simulink model "Lora_os_all_16M64M_bw500sf12"  (R2022b)
settings: Solver=FixedStepDiscrete  StartTime=0.0  StopTime=0.06  RelTol=1e-3
undefined symbols (not defined in the file or in its folder): cr, crc, fs, has_header, ldr, payload, preamble_len, sf
libraries: hdlsllib x4, simulink x2
settings Model: DataTypeOverride=Off  Creator=28627  LastModifiedBy=X_Ditto
settings SolverCC: AlgebraicLoopSolver=TrustRegion
settings DataIOCC: SaveOutput=off  SaveTime=off
settings OptimizationCC: BlockReduction=off  ConditionallyExecuteInputs=off  DefaultParameterBehavior=Inlined
settings DebuggingCC: AlgebraicLoopMsg=error  SingleTaskRateTransMsg=error  UnconnectedInputMsg=warning  UnconnectedOutputMsg=warning  UnconnectedLineMsg=warning  StrictBusMsg=ErrorOnBusTreatedAsVector  SFMachineParentedDataDiag=warning  ArithmeticOperatorsInVariantConditions=warning
settings HardwareCC: ProdBitPerPointer=32  ProdBitPerSizeT=32  ProdBitPerPtrDiffT=32  ProdLargestAtomicFloat=None  ProdIntDivRoundTo=Undefined  ProdEndianess=Unspecified  ProdWordSize=32  ProdHWDeviceType=ASIC/FPGA->ASIC/FPGA  ProdEqTarget=off
settings ModelReferenceCC: EnableRefExpFcnMdlSchedulingChecks=on
settings SFSimCC: SimUseLocalCustomCode=off  CustomCodeUndefinedFunction=UseInterfaceOnly
settings RTWCC: RTWUseLocalCustomCode=off
settings CodeAppCC: StateflowObjectComments=on
settings GRTTargetCC: TargetLangStandard=C89/C90 (ANSI)

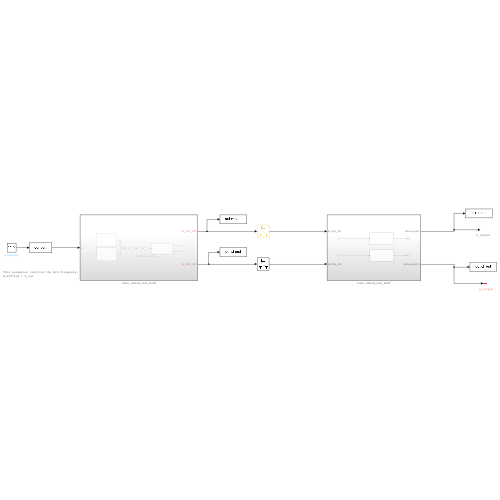
[thumbnail: Simulink's stored preview of the top-level diagram]
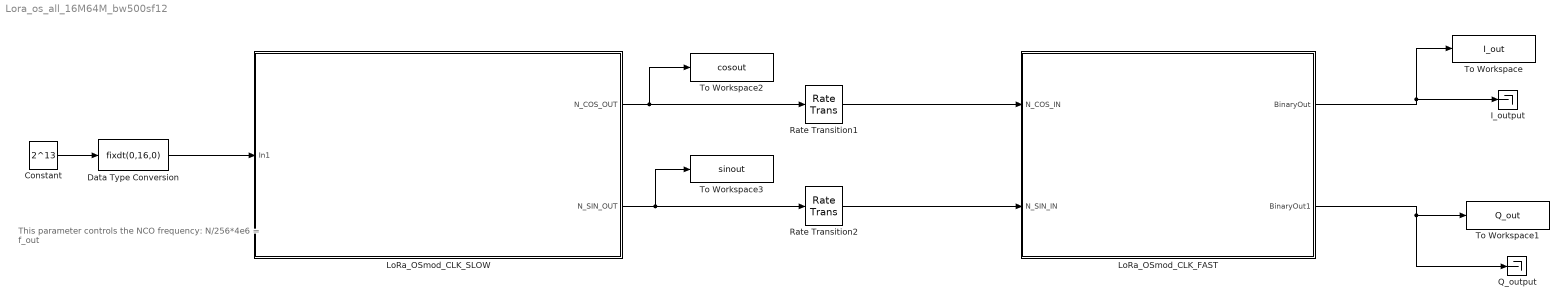
== system Lora_os_all_16M64M_bw500sf12 ==
  note: This parameter controls the NCO frequency:
      | N/256*4e6 = f_out
  Constant : Constant  Value=2^13  SampleTime=1/16e6
  Data Type Conversion : DataTypeConversion  OutDataTypeStr=fixdt(0,16,0)  SaturateOnIntegerOverflow=off  RndMeth=Floor
  I_output : Terminator
  LoRa_OSmod_CLK_FAST : Subsystem
  LoRa_OSmod_CLK_SLOW : Subsystem
  Q_output : Terminator
  Rate Transition1 : RateTransition  OutPortSampleTime=1/64e6
  Rate Transition2 : RateTransition  OutPortSampleTime=1/64e6
  To Workspace : ToWorkspace  VariableName=I_out  SampleTime=-1
      settings: Save2DSignal=2-D array (concatenate along first dimension)
  To Workspace1 : ToWorkspace  VariableName=Q_out  SampleTime=-1
      settings: Save2DSignal=2-D array (concatenate along first dimension)
  To Workspace2 : ToWorkspace  VariableName=cosout  SampleTime=-1
      settings: Save2DSignal=2-D array (concatenate along first dimension)
  To Workspace3 : ToWorkspace  VariableName=sinout  SampleTime=-1
      settings: Save2DSignal=2-D array (concatenate along first dimension)
  wires:
  Constant/1 -> Data Type Conversion/1
  Data Type Conversion/1 -> LoRa_OSmod_CLK_SLOW/1(In1)
  LoRa_OSmod_CLK_FAST/1(BinaryOut) -> To Workspace/1, I_output/1
  LoRa_OSmod_CLK_FAST/2(BinaryOut1) -> Q_output/1, To Workspace1/1
  LoRa_OSmod_CLK_SLOW/1(N_COS_OUT) -> To Workspace2/1, Rate Transition1/1
  LoRa_OSmod_CLK_SLOW/2(N_SIN_OUT) -> To Workspace3/1, Rate Transition2/1
  Rate Transition1/1 -> LoRa_OSmod_CLK_FAST/1(N_COS_IN)
  Rate Transition2/1 -> LoRa_OSmod_CLK_FAST/2(N_SIN_IN)

== system Lora_os_all_16M64M_bw500sf12/LoRa_OSmod_CLK_FAST ==
  N_COS_IN : Inport
  N_SIN_IN : Inport  Port=2
  DeltaMod : Subsystem
  DeltaMod1 : Subsystem
  BinaryOut : Outport
  BinaryOut1 : Outport  Port=2
  wires:
  N_SIN_IN/1 -> DeltaMod1/1(WaveIn)
  N_COS_IN/1 -> DeltaMod/1(WaveIn)
  DeltaMod/1(BinaryOut) -> BinaryOut/1
  DeltaMod1/1(BinaryOut) -> BinaryOut1/1

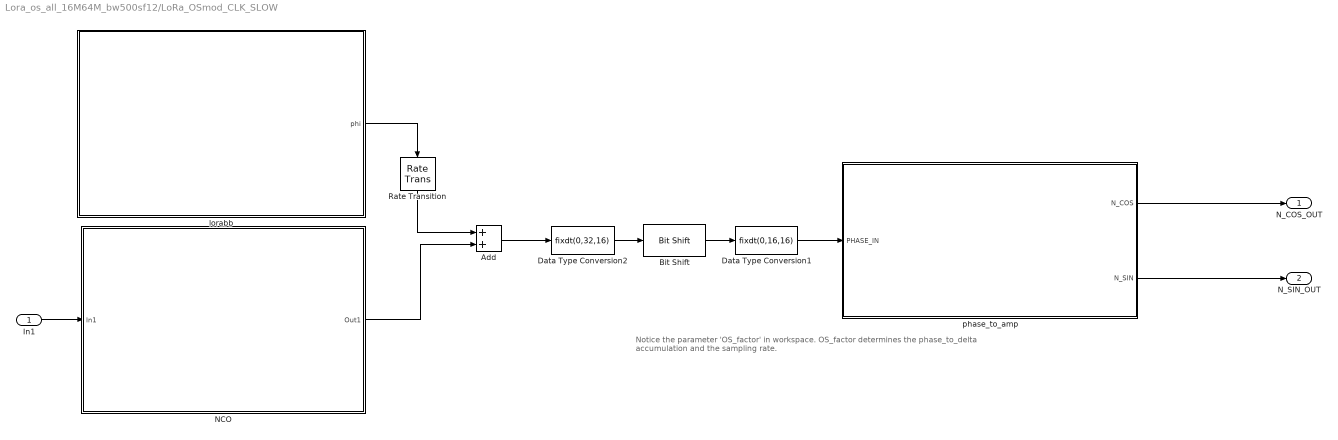
== system Lora_os_all_16M64M_bw500sf12/LoRa_OSmod_CLK_SLOW ==
  note: Notice the parameter 'OS_factor' in workspace. OS_factor determines the phase_to_delta accumulation and the sampling rate.
  In1 : Inport
  Add : Sum
  Bit Shift : hdlsllib/Logic and Bit Operations/Bit Shift  mode=Shift Right Logical  N=16
  Data Type Conversion1 : DataTypeConversion  OutDataTypeStr=fixdt(0,16,16)  SaturateOnIntegerOverflow=off  RndMeth=Floor
  Data Type Conversion2 : DataTypeConversion  OutDataTypeStr=fixdt(0,32,16)  SaturateOnIntegerOverflow=off  RndMeth=Floor
  NCO : Subsystem
  Rate Transition : RateTransition
  lorabb : Subsystem
  phase_to_amp : Subsystem
  N_COS_OUT : Outport
  N_SIN_OUT : Outport  Port=2
  wires:
  Data Type Conversion2/1 -> Bit Shift/1
  Data Type Conversion1/1 -> phase_to_amp/1(PHASE_IN)
  lorabb/1(phi) -> Rate Transition/1
  Rate Transition/1 -> Add/1
  Bit Shift/1 -> Data Type Conversion1/1
  Add/1 -> Data Type Conversion2/1
  NCO/1(Out1) -> Add/2
  In1/1 -> NCO/1(In1)
  phase_to_amp/1(N_COS) -> N_COS_OUT/1
  phase_to_amp/2(N_SIN) -> N_SIN_OUT/1

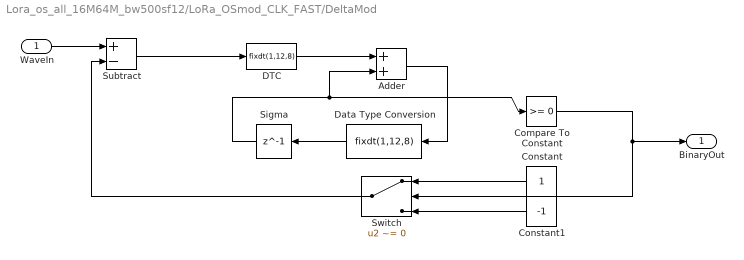
== system Lora_os_all_16M64M_bw500sf12/LoRa_OSmod_CLK_FAST/DeltaMod ==
  WaveIn : Inport
  Adder : Sum
  Compare To Constant : simulink/Logic and Bit Operations/Compare To Constant  relop=>=  const=0  OutDataTypeStr=boolean
  Constant : Constant  OutDataTypeStr=fixdt(1,10,8)  SampleTime=-1
  Constant1 : Constant  Value=-1  OutDataTypeStr=fixdt(1,10,8)  SampleTime=-1
  DTC : DataTypeConversion  OutDataTypeStr=fixdt(1,12,8)  RndMeth=Floor
  Data Type Conversion : DataTypeConversion  OutDataTypeStr=fixdt(1,12,8)  SaturateOnIntegerOverflow=off  RndMeth=Floor
  Sigma : Delay  DelayLength=1
  Subtract : Sum  Inputs=+-
  Switch : Switch  Criteria=u2 ~= 0  SaturateOnIntegerOverflow=off  InputSameDT=off
  BinaryOut : Outport
  wires:
  WaveIn/1 -> Subtract/1
  Adder/1 -> Data Type Conversion/1
  Sigma/1 -> Adder/2, Compare To Constant/1
  Constant/1 -> Switch/1
  Constant1/1 -> Switch/3
  Compare To Constant/1 -> BinaryOut/1, Switch/2
  Switch/1 -> Subtract/2
  DTC/1 -> Adder/1
  Data Type Conversion/1 -> Sigma/1
  Subtract/1 -> DTC/1

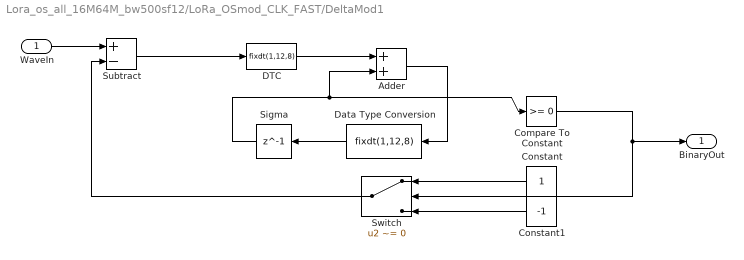
== system Lora_os_all_16M64M_bw500sf12/LoRa_OSmod_CLK_FAST/DeltaMod1 ==
  WaveIn : Inport
  Adder : Sum
  Compare To Constant : simulink/Logic and Bit Operations/Compare To Constant  relop=>=  const=0  OutDataTypeStr=boolean
  Constant : Constant  OutDataTypeStr=fixdt(1,10,8)  SampleTime=-1
  Constant1 : Constant  Value=-1  OutDataTypeStr=fixdt(1,10,8)  SampleTime=-1
  DTC : DataTypeConversion  OutDataTypeStr=fixdt(1,12,8)  RndMeth=Floor
  Data Type Conversion : DataTypeConversion  OutDataTypeStr=fixdt(1,12,8)  SaturateOnIntegerOverflow=off  RndMeth=Floor
  Sigma : Delay  DelayLength=1
  Subtract : Sum  Inputs=+-
  Switch : Switch  Criteria=u2 ~= 0  SaturateOnIntegerOverflow=off  InputSameDT=off
  BinaryOut : Outport
  wires:
  WaveIn/1 -> Subtract/1
  Adder/1 -> Data Type Conversion/1
  Sigma/1 -> Adder/2, Compare To Constant/1
  Constant/1 -> Switch/1
  Constant1/1 -> Switch/3
  Compare To Constant/1 -> BinaryOut/1, Switch/2
  Switch/1 -> Subtract/2
  DTC/1 -> Adder/1
  Data Type Conversion/1 -> Sigma/1
  Subtract/1 -> DTC/1

== system Lora_os_all_16M64M_bw500sf12/LoRa_OSmod_CLK_SLOW/NCO ==
  In1 : Inport
  Add : Sum
  Bit Slice : hdlsllib/Logic and Bit Operations/Bit Slice  lidx=15  ridx=0
  Delay : Delay  DelayLength=1
  Out1 : Outport
  wires:
  Delay/1 -> Add/2, Out1/1
  In1/1 -> Add/1
  Add/1 -> Bit Slice/1
  Bit Slice/1 -> Delay/1

== system Lora_os_all_16M64M_bw500sf12/LoRa_OSmod_CLK_SLOW/lorabb ==
  Encode : Subsystem
  Modulate : Subsystem
  phi : Outport
  wires:
  Encode/1(symbols) -> Modulate/1(data_symbols)
  Encode/2(symbols_rdy) -> Modulate/2(ready)
  Encode/3(sym_num) -> Modulate/3(sym_num)
  Modulate/1(phi) -> phi/1

== system Lora_os_all_16M64M_bw500sf12/LoRa_OSmod_CLK_SLOW/phase_to_amp ==
  PHASE_IN : Inport
  Cosine HDL Optimized : hdlsllib/Lookup Tables/Cosine HDL Optimized  OutputFormula=cos(2*pi*u)  NumDataPoints=256  TableDataTypeStr=fixdt(0,9,8)  SimulateLUTROMDelay=off
  Sine HDL Optimized : hdlsllib/Lookup Tables/Cosine HDL Optimized  OutputFormula=sin(2*pi*u)  NumDataPoints=256  TableDataTypeStr=fixdt(0,9,8)  SimulateLUTROMDelay=off
      settings: LibrarySourceBlock=|
      | hdlsllib/Lookup
      | Tables/Sine
      | HDL Optimized
  N_COS : Outport
  N_SIN : Outport  Port=2
  wires:
  PHASE_IN/1 -> Sine HDL Optimized/1, Cosine HDL Optimized/1
  Cosine HDL Optimized/1 -> N_COS/1
  Sine HDL Optimized/1 -> N_SIN/1

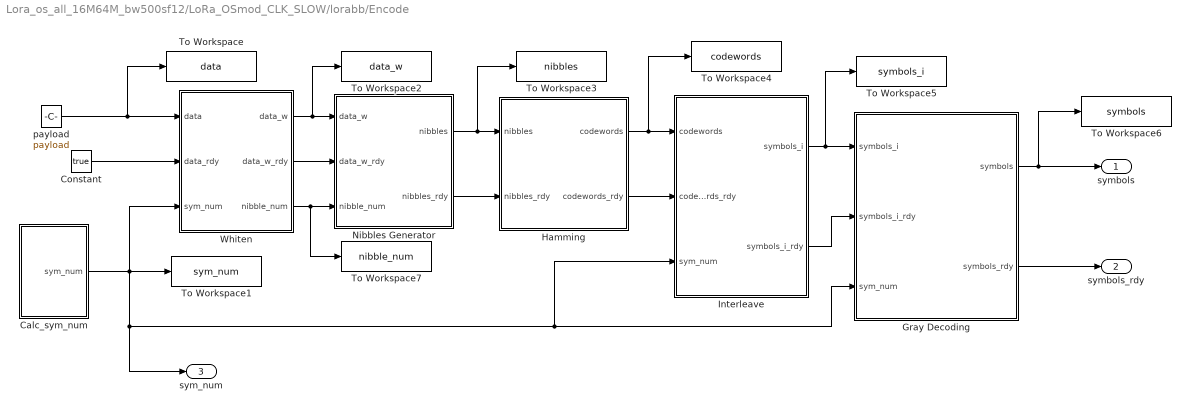
== system Lora_os_all_16M64M_bw500sf12/LoRa_OSmod_CLK_SLOW/lorabb/Encode ==
  Calc_sym_num : Subsystem
  Constant : Constant  Value=true  OutDataTypeStr=boolean  SampleTime=1/fs
  Gray Decoding : Subsystem
  Hamming : Subsystem
  Interleave : Subsystem
  Nibbles Generator : Subsystem
  To Workspace : ToWorkspace  VariableName=data  SampleTime=-1
  To Workspace1 : ToWorkspace  VariableName=sym_num  SampleTime=-1
  To Workspace2 : ToWorkspace  VariableName=data_w  SampleTime=-1
  To Workspace3 : ToWorkspace  VariableName=nibbles  SampleTime=-1
  To Workspace4 : ToWorkspace  VariableName=codewords  SampleTime=-1
  To Workspace5 : ToWorkspace  VariableName=symbols_i  SampleTime=-1
  To Workspace6 : ToWorkspace  VariableName=symbols  SampleTime=-1
  To Workspace7 : ToWorkspace  VariableName=nibble_num  SampleTime=-1
  Whiten : Subsystem
  payload : Constant  Value=payload  OutDataTypeStr=uint8  SampleTime=1/fs
  symbols : Outport
  symbols_rdy : Outport  Port=2
  sym_num : Outport  Port=3
  wires:
  Interleave/1(symbols_i) -> To Workspace5/1, Gray Decoding/1(symbols_i)
  Gray Decoding/1(symbols) -> To Workspace6/1, symbols/1
  Whiten/3(nibble_num) -> To Workspace7/1, Nibbles Generator/3(nibble_num)
  Whiten/1(data_w) -> Nibbles Generator/1(data_w), To Workspace2/1
  Nibbles Generator/1(nibbles) -> Hamming/1(nibbles), To Workspace3/1
  Hamming/1(codewords) -> To Workspace4/1, Interleave/1(codewords)
  Calc_sym_num/1(sym_num) -> Whiten/3(sym_num), To Workspace1/1, sym_num/1, Gray Decoding/3(sym_num), Interleave/3(sym_num)
  payload/1 -> Whiten/1(data), To Workspace/1
  Constant/1 -> Whiten/2(data_rdy)
  Whiten/2(data_w_rdy) -> Nibbles Generator/2(data_w_rdy)
  Nibbles Generator/2(nibbles_rdy) -> Hamming/2(nibbles_rdy)
  Hamming/2(codewords_rdy) -> Interleave/2(codewords_rdy)
  Interleave/2(symbols_i_rdy) -> Gray Decoding/2(symbols_i_rdy)
  Gray Decoding/2(symbols_rdy) -> symbols_rdy/1

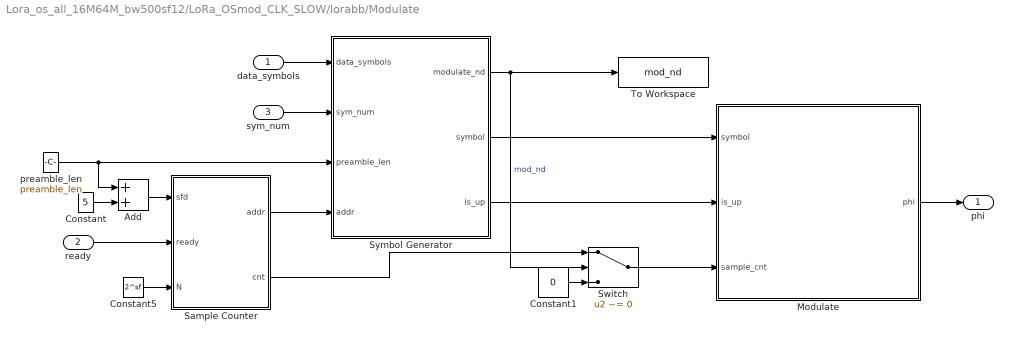
== system Lora_os_all_16M64M_bw500sf12/LoRa_OSmod_CLK_SLOW/lorabb/Modulate ==
  data_symbols : Inport
  ready : Inport  Port=2
  sym_num : Inport  Port=3
  Add : Sum  OutDataTypeStr=uint16
  Constant : Constant  Value=5  OutDataTypeStr=uint16  SampleTime=1/fs
  Constant1 : Constant  Value=0  OutDataTypeStr=uint16  SampleTime=1/fs
  Constant5 : Constant  Value=2^sf  OutDataTypeStr=uint16  SampleTime=1/fs
  Modulate : Subsystem
  Sample Counter : MATLAB Function  TreatAsAtomicUnit=on
  Switch : Switch  Criteria=u2 ~= 0  SaturateOnIntegerOverflow=off  InputSameDT=off
  Symbol Generator : MATLAB Function  TreatAsAtomicUnit=on
  To Workspace : ToWorkspace  VariableName=mod_nd  SampleTime=-1
      settings: Save2DSignal=2-D array (concatenate along first dimension)
  preamble_len : Constant  Value=preamble_len  OutDataTypeStr=uint16  SampleTime=1/fs
  phi : Outport
  wires:
  data_symbols/1 -> Symbol Generator/1(data_symbols)
  Symbol Generator/2(symbol) -> Modulate/1(symbol)
  Constant5/1 -> Sample Counter/3(N)
  Sample Counter/2(cnt) -> Switch/1
  sym_num/1 -> Symbol Generator/2(sym_num)
  preamble_len/1 -> Add/1, Symbol Generator/3(preamble_len)
  Sample Counter/1(addr) -> Symbol Generator/4(addr)
  Add/1 -> Sample Counter/1(sfd)
  Constant/1 -> Add/2
  Symbol Generator/3(is_up) -> Modulate/2(is_up)
  Symbol Generator/1(modulate_nd) -> To Workspace/1, Switch/2  "mod_nd"
  ready/1 -> Sample Counter/2(ready)
  Constant1/1 -> Switch/3
  Switch/1 -> Modulate/3(sample_cnt)
  Modulate/1(phi) -> phi/1

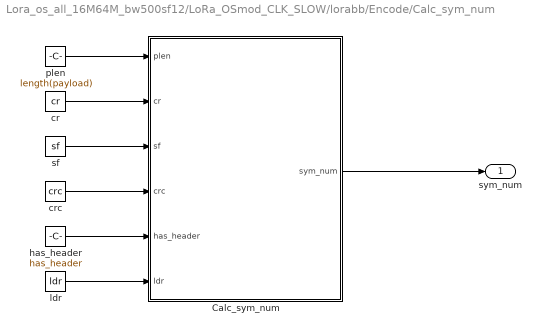
== system Lora_os_all_16M64M_bw500sf12/LoRa_OSmod_CLK_SLOW/lorabb/Encode/Calc_sym_num ==
  Calc_sym_num : MATLAB Function  TreatAsAtomicUnit=on
  cr : Constant  Value=cr  VectorParams1D=off  OutDataTypeStr=uint8  SampleTime=1/fs
  crc : Constant  Value=crc  VectorParams1D=off  OutDataTypeStr=uint8  SampleTime=1/fs
  has_header : Constant  Value=has_header  VectorParams1D=off  OutDataTypeStr=uint8  SampleTime=1/fs
  ldr : Constant  Value=ldr  VectorParams1D=off  OutDataTypeStr=uint8  SampleTime=1/fs
  plen : Constant  Value=length(payload)  VectorParams1D=off  OutDataTypeStr=uint8  SampleTime=1/fs
  sf : Constant  Value=sf  VectorParams1D=off  OutDataTypeStr=uint8  SampleTime=1/fs
  sym_num : Outport
  wires:
  sf/1 -> Calc_sym_num/3(sf)
  ldr/1 -> Calc_sym_num/6(ldr)
  has_header/1 -> Calc_sym_num/5(has_header)
  crc/1 -> Calc_sym_num/4(crc)
  Calc_sym_num/1(sym_num) -> sym_num/1
  cr/1 -> Calc_sym_num/2(cr)
  plen/1 -> Calc_sym_num/1(plen)

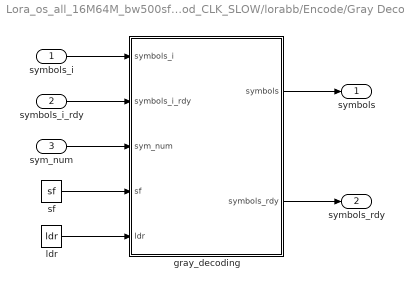
== system Lora_os_all_16M64M_bw500sf12/LoRa_OSmod_CLK_SLOW/lorabb/Encode/Gray Decoding ==
  symbols_i : Inport
  symbols_i_rdy : Inport  Port=2
  sym_num : Inport  Port=3
  gray_decoding : MATLAB Function  TreatAsAtomicUnit=on
  ldr : Constant  Value=ldr  OutDataTypeStr=uint8  SampleTime=1/fs
  sf : Constant  Value=sf  OutDataTypeStr=uint8  SampleTime=1/fs
  symbols : Outport
  symbols_rdy : Outport  Port=2
  wires:
  ldr/1 -> gray_decoding/5(ldr)
  sf/1 -> gray_decoding/4(sf)
  symbols_i/1 -> gray_decoding/1(symbols_i)
  gray_decoding/1(symbols) -> symbols/1
  symbols_i_rdy/1 -> gray_decoding/2(symbols_i_rdy)
  gray_decoding/2(symbols_rdy) -> symbols_rdy/1
  sym_num/1 -> gray_decoding/3(sym_num)

== system Lora_os_all_16M64M_bw500sf12/LoRa_OSmod_CLK_SLOW/lorabb/Encode/Hamming ==
  nibbles : Inport
  nibbles_rdy : Inport  Port=2
  Constant : Constant  Value=sf  OutDataTypeStr=uint8  SampleTime=1/fs
  Constant1 : Constant  Value=cr  OutDataTypeStr=uint8  SampleTime=1/fs
  hamming : MATLAB Function  TreatAsAtomicUnit=on
  codewords : Outport
  codewords_rdy : Outport  Port=2
  wires:
  hamming/1(codewords) -> codewords/1
  nibbles/1 -> hamming/3(nibbles)
  Constant/1 -> hamming/1(sf)
  Constant1/1 -> hamming/2(cr)
  nibbles_rdy/1 -> hamming/4(nibbles_rdy)
  hamming/2(codewords_rdy) -> codewords_rdy/1

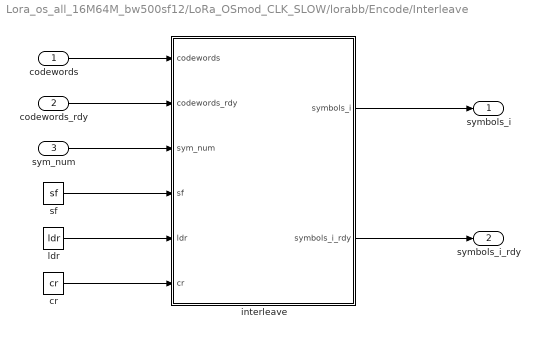
== system Lora_os_all_16M64M_bw500sf12/LoRa_OSmod_CLK_SLOW/lorabb/Encode/Interleave ==
  codewords : Inport
  codewords_rdy : Inport  Port=2
  sym_num : Inport  Port=3
  cr : Constant  Value=cr  OutDataTypeStr=uint8  SampleTime=1/fs
  interleave : MATLAB Function  TreatAsAtomicUnit=on
  ldr : Constant  Value=ldr  OutDataTypeStr=uint8  SampleTime=1/fs
  sf : Constant  Value=sf  OutDataTypeStr=uint8  SampleTime=1/fs
  symbols_i : Outport
  symbols_i_rdy : Outport  Port=2
  wires:
  sf/1 -> interleave/4(sf)
  ldr/1 -> interleave/5(ldr)
  cr/1 -> interleave/6(cr)
  interleave/1(symbols_i) -> symbols_i/1
  codewords/1 -> interleave/1(codewords)
  codewords_rdy/1 -> interleave/2(codewords_rdy)
  interleave/2(symbols_i_rdy) -> symbols_i_rdy/1
  sym_num/1 -> interleave/3(sym_num)

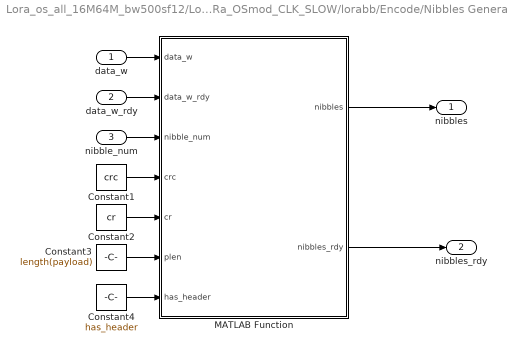
== system Lora_os_all_16M64M_bw500sf12/LoRa_OSmod_CLK_SLOW/lorabb/Encode/Nibbles Generator ==
  data_w : Inport
  data_w_rdy : Inport  Port=2
  nibble_num : Inport  Port=3
  Constant1 : Constant  Value=crc  OutDataTypeStr=uint8  SampleTime=1/fs
  Constant2 : Constant  Value=cr  OutDataTypeStr=uint8  SampleTime=1/fs
  Constant3 : Constant  Value=length(payload)  OutDataTypeStr=uint8  SampleTime=1/fs
  Constant4 : Constant  Value=has_header  OutDataTypeStr=uint8  SampleTime=1/fs
  MATLAB Function : MATLAB Function  TreatAsAtomicUnit=on
  nibbles : Outport
  nibbles_rdy : Outport  Port=2
  wires:
  nibble_num/1 -> MATLAB Function/3(nibble_num)
  data_w/1 -> MATLAB Function/1(data_w)
  Constant1/1 -> MATLAB Function/4(crc)
  Constant2/1 -> MATLAB Function/5(cr)
  Constant3/1 -> MATLAB Function/6(plen)
  Constant4/1 -> MATLAB Function/7(has_header)
  MATLAB Function/1(nibbles) -> nibbles/1
  data_w_rdy/1 -> MATLAB Function/2(data_w_rdy)
  MATLAB Function/2(nibbles_rdy) -> nibbles_rdy/1

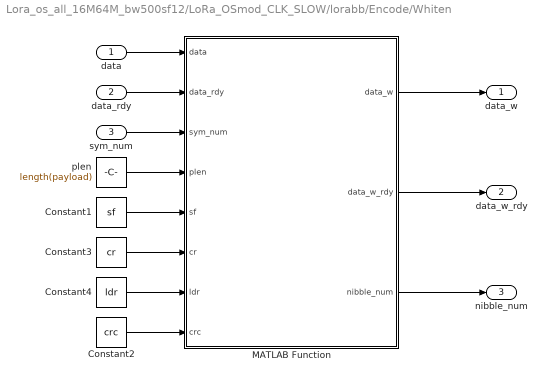
== system Lora_os_all_16M64M_bw500sf12/LoRa_OSmod_CLK_SLOW/lorabb/Encode/Whiten ==
  data : Inport
  data_rdy : Inport  Port=2
  sym_num : Inport  Port=3
  Constant1 : Constant  Value=sf  OutDataTypeStr=uint8  SampleTime=1/fs
  Constant2 : Constant  Value=crc  OutDataTypeStr=uint8  SampleTime=1/fs
  Constant3 : Constant  Value=cr  OutDataTypeStr=uint8  SampleTime=1/fs
  Constant4 : Constant  Value=ldr  OutDataTypeStr=uint8  SampleTime=1/fs
  MATLAB Function : MATLAB Function  TreatAsAtomicUnit=on
  plen : Constant  Value=length(payload)  OutDataTypeStr=uint8  SampleTime=1/fs
  data_w : Outport
  data_w_rdy : Outport  Port=2
  nibble_num : Outport  Port=3
  wires:
  MATLAB Function/1(data_w) -> data_w/1
  Constant4/1 -> MATLAB Function/7(ldr)
  Constant1/1 -> MATLAB Function/5(sf)
  sym_num/1 -> MATLAB Function/3(sym_num)
  data/1 -> MATLAB Function/1(data)
  plen/1 -> MATLAB Function/4(plen)
  Constant3/1 -> MATLAB Function/6(cr)
  MATLAB Function/3(nibble_num) -> nibble_num/1
  Constant2/1 -> MATLAB Function/8(crc)
  data_rdy/1 -> MATLAB Function/2(data_rdy)
  MATLAB Function/2(data_w_rdy) -> data_w_rdy/1

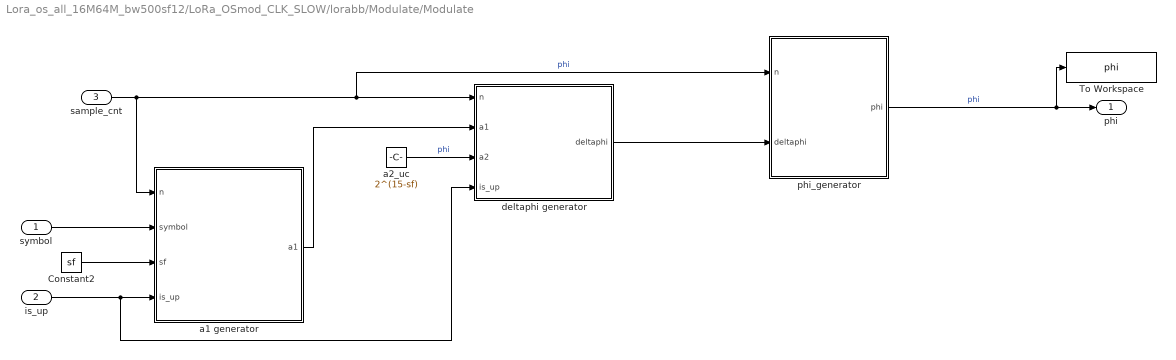
== system Lora_os_all_16M64M_bw500sf12/LoRa_OSmod_CLK_SLOW/lorabb/Modulate/Modulate ==
  symbol : Inport
  is_up : Inport  Port=2
  sample_cnt : Inport  Port=3
  Constant2 : Constant  Value=sf  OutDataTypeStr=uint16  SampleTime=1/fs
  To Workspace : ToWorkspace  VariableName=phi  SampleTime=-1
      settings: Save2DSignal=2-D array (concatenate along first dimension)
  a1 generator : MATLAB Function  TreatAsAtomicUnit=on
  a2_uc : Constant  Value=2^(15-sf)  OutDataTypeStr=uint16  SampleTime=1/fs
  deltaphi generator : MATLAB Function  TreatAsAtomicUnit=on
  phi_generator : MATLAB Function  TreatAsAtomicUnit=on
  phi : Outport
  wires:
  symbol/1 -> a1 generator/2(symbol)
  Constant2/1 -> a1 generator/3(sf)
  a1 generator/1(a1) -> deltaphi generator/2(a1)
  phi_generator/1(phi) -> phi/1, To Workspace/1  "phi"
  deltaphi generator/1(deltaphi) -> phi_generator/2(deltaphi)
  is_up/1 -> deltaphi generator/4(is_up), a1 generator/4(is_up)
  sample_cnt/1 -> phi_generator/1(n), deltaphi generator/1(n), a1 generator/1(n)  "phi"
  a2_uc/1 -> deltaphi generator/3(a2)  "phi"

== matlab function Lora_os_all_16M64M_bw500sf12/LoRa_OSmod_CLK_SLOW/lorabb/Encode/Gray Decoding/gray_decoding ==
  data: symbols_i input; symbols output; symbols_i_rdy input; sym_num input; sf input; ldr input; symbols_rdy output
% function [symbols,symbols_rdy] = gray_decoding(symbols_i,symbols_i_rdy,sf,ldr)
% symbols = fi(zeros(1,64),0,16,0);
% for k = 1:64
%     num = symbols_i(k);
%     mask = bitshift(num, -1);
%     for m=1:16
%         num = bitxor(num, mask);
%         mask = bitshift(mask, -1);
%     end
%     if k <= 8 || fi(ldr,0,8,0)==fi(1,0,8,0)
% %       symbols(k) = mod(num * 4 + 1, 2^sf);
%         tmp = bitsliceget(fi(bitshift(num,2),0,16,0)+fi(1,0,16,0),16,1);
%         for m = 16:-1:1
%             if fi(m,0,8,0)<bitsliceget(fi(sf,0,8,0)+fi(1,0,8,0),8,1)
%                 symbols(k) = bitsliceget(fi(symbols(k),0,16,0)+fi(symbols(k),0,16,0)+fi(bitget(tmp,m),0,16,0),16,1);
%             end
%         end
%     else
% %       symbols(k) = mod(num + 1, 2^sf);
%         tmp = bitsliceget(fi(num,0,16,0)+fi(1,0,16,0),16,1);
%         for m = 16:-1:1
%             if fi(m,0,8,0)<bitsliceget(fi(sf,0,8,0)+fi(1,0,8,0),8,1)
%                 symbols(k) = bitsliceget(fi(symbols(k),0,16,0)+fi(symbols(k),0,16,0)+fi(bitget(tmp,m),0,16,0),16,1);
%             end
%         end
%     end
% end
% symbols_rdy=symbols_i_rdy;
function [symbols,symbols_rdy] = gray_decoding(symbols_i,symbols_i_rdy,sym_num,sf,ldr)
persistent p_idx ...
           i_idx ...
           b_idx ...
           num ...
           mask ...
           tmp_symbols
if isempty(p_idx)
    p_idx = fi(1,0,8,0);
end
if isempty(i_idx)
    i_idx = fi(0,0,8,0);
end
if isempty(b_idx)
    b_idx = fi(1,0,8,0);
end
if isempty(num)
    num = fi(0,0,16,0);
end
if isempty(mask)
    mask = fi(0,0,16,0);
end
if isempty(tmp_symbols)
    tmp_symbols = fi(zeros(1,64),0,16,0);
end

if symbols_i_rdy==true
    if p_idx<=fi(sym_num,0,8,0)
        if i_idx==fi(0,0,8,0)
            num = fi(symbols_i(p_idx),0,16,0);
            mask = bitshift(num, -1);
            i_idx=fi(1,0,8,0);
        elseif i_idx<=fi(16,0,8,0)
            num = bitxor(num, mask);
            mask = bitshift(mask, -1);
            i_idx=fi(i_idx+1,0,8,0);
        else
            if p_idx <= fi(8,0,8,0) || fi(ldr,0,8,0)==fi(1,0,8,0)
                tmp = bitsliceget(fi(bitshift(num,2),0,16,0)+fi(1,0,16,0),16,1);
                if fi(b_idx,0,8,0)<bitsliceget(fi(sf,0,8,0)+fi(1,0,8,0),8,1)
                    tmp_symbols(p_idx) = bitsliceget(fi(tmp_symbols(p_idx),0,16,0)+fi(tmp_symbols(p_idx),0,16,0)+fi(bitget(tmp,sf+1-b_idx),0,16,0),16,1);
                    b_idx=fi(b_idx+1,0,8,0);
                else
                    p_idx=fi(p_idx+1,0,8,0);
                    i_idx=fi(0,0,8,0);
                    b_idx=fi(1,0,8,0);
                end
            else
                tmp = bitsliceget(fi(num,0,16,0)+fi(1,0,16,0),16,1);
                if fi(b_idx,0,8,0)<bitsliceget(fi(sf,0,8,0)+fi(1,0,8,0),8,1)
                    tmp_symbols(p_idx) = bitsliceget(fi(tmp_symbols(p_idx),0,16,0)+fi(tmp_symbols(p_idx),0,16,0)+fi(bitget(tmp,sf+1-b_idx),0,16,0),16,1);
                    b_idx=fi(b_idx+1,0,8,0);
                else
                    p_idx=fi(p_idx+1,0,8,0);
                    i_idx=fi(0,0,8,0);
                    b_idx=fi(1,0,8,0);
                end
            end
        end
        symbols=fi(zeros(1,64),0,16,0);
        symbols_rdy=false;
    else
        symbols=tmp_symbols;
        symbols_rdy=true;
    end
else
    symbols=fi(zeros(1,64),0,16,0);
    symbols_rdy=false;
end

== matlab function Lora_os_all_16M64M_bw500sf12/LoRa_OSmod_CLK_SLOW/lorabb/Modulate/Modulate/a1 generator ==
  data: n input; symbol input; a1 output; sf input; is_up input
function a1 = a1_generator(n,symbol,sf,is_up)
if is_up==true
    if n+symbol<=2^sf
        a1=bitsliceget(bitshift(fi(symbol,0,32,0),16-sf),16,1);
    else
        a1=bitsliceget(bitshift(fi(1,0,32,0),16-sf),16,1);
    end
else
    if n+symbol<=2^sf
        a1=bitsliceget(fi(fi(65536,0,32,0)-bitshift(fi(symbol,0,32,0),16-sf),0,32,0),16,1);
    else
        a1=bitsliceget(fi(fi(65536,0,32,0)-bitshift(fi(1,0,32,0),16-sf),0,32,0),16,1);
    end
end

== matlab function Lora_os_all_16M64M_bw500sf12/LoRa_OSmod_CLK_SLOW/lorabb/Modulate/Modulate/deltaphi generator ==
  data: n input; a1 input; deltaphi output; a2 input; is_up input
function deltaphi  = deltaphi_gen(n,a1,a2,is_up)
persistent flag...
           last_a1
if isempty(flag)
    flag=fi(0,0,16,0);
end
if isempty(last_a1)
    last_a1=fi(0,0,16,0);
end
if fi(n,0,16,0)==fi(0,0,16,0)
    deltaphi=fi(0,0,16,0);
    flag=fi(0,0,16,0);
    last_a1=fi(a1,0,16,0);
else
    if flag==fi(0,0,16,0) && last_a1~=fi(a1,0,16,0)
        flag=fi(n,0,16,0);
        if is_up
            if a1>=a2
                deltaphi=fi(a1-a2,0,16,0);
            else
                deltaphi=fi(fi(65535,0,16,0)-a2+a1,0,16,0);
            end
        else
            deltaphi=bitsliceget(fi(a1,0,32,0)+fi(a2,0,32,0),16,1);
        end
    else
        if is_up
            deltaphi=bitsliceget(fi(fi(a1,0,32,0)+fi(a2,0,32,0)*fi((2*(n-flag)-1),0,32,0),0,32,0),16,1);
        else
            if a1>a2*(2*(n-flag)-1)
                deltaphi=bitsliceget(fi(fi(a1,0,32,0)-fi(a2,0,32,0)*fi((2*(n-flag)-1),0,32,0),0,32,0),16,1);
            else
                deltaphi=bitsliceget(fi(fi(2^16,0,32,0)+fi(a1,0,32,0)-fi(a2,0,32,0)*fi((2*(n-flag)-1),0,32,0),0,32,0),16,1);
            end
        end
    end
    if deltaphi>fi(32767,0,16,0)
        deltaphi=fi(deltaphi-fi(32768,0,16,0),0,16,0);
    else
        deltaphi=fi(deltaphi+fi(32768,0,16,0),0,16,0);
    end
end

== matlab function Lora_os_all_16M64M_bw500sf12/LoRa_OSmod_CLK_SLOW/lorabb/Modulate/Modulate/phi_generator ==
  data: n input; deltaphi input; phi output
function phi = phi_generator(n,deltaphi)
persistent last_phi
if isempty(last_phi)
    last_phi=fi(0,0,16,0);
end
phi=bitsliceget(fi(fi(last_phi,0,32,0)+fi(deltaphi,0,32,0),0,32,0),16,1);

if fi(n,0,32,0)==fi(0,0,32,0)
    phi=fi(0,0,16,0);
end
last_phi=phi;

== matlab function Lora_os_all_16M64M_bw500sf12/LoRa_OSmod_CLK_SLOW/lorabb/Modulate/Sample Counter ==
  data: sfd input; addr output; ready input; cnt output; N input
function [addr,cnt] = samp_cnt(sfd,ready,N)
% cnt [0,samp-1]
% addr [1,end]

persistent last_cnt...
           last_addr
if isempty(last_cnt)
    last_cnt=fi(N-1,0,16,0);
end
if isempty(last_addr)
    last_addr=fi(0,0,16,0);
end

addr=last_addr;
if ready==true
    cnt=fi(last_cnt+fi(1,0,16,0),0,16,0);
    if (cnt==N)|| (addr==sfd && cnt==fi(bitshift(N,-2),0,16,0))
        cnt=fi(0,0,16,0);
        addr=fi(last_addr+fi(1,0,16,0),0,16,0);
        last_addr=addr;
    end
    last_cnt=cnt;
else
    last_cnt=fi(N-1,0,16,0);
    last_addr=fi(0,0,16,0);
    cnt=fi(0,0,16,0);
end

== matlab function Lora_os_all_16M64M_bw500sf12/LoRa_OSmod_CLK_SLOW/lorabb/Encode/Nibbles Generator/MATLAB Function ==
  data: data_w input; data_w_rdy input; nibbles output; nibble_num input; crc input; cr input; plen input; has_header input; nibbles_rdy output
function [nibbles,nibbles_rdy]=nibbles(data_w,data_w_rdy,nibble_num,crc,cr,plen,has_header)
persistent idx...
           w_idx...
           tmp_nibbles
if isempty(idx)
    idx=fi(1,0,8,0);
end
if isempty(w_idx)
    w_idx=fi(1,0,8,0);
end
if isempty(tmp_nibbles)
    tmp_nibbles=fi(zeros(1,16),0,8,0);
end

if data_w_rdy==true
    if fi(has_header,0,8,0)==fi(1,0,8,0)
        header_nibbles = fi(zeros(1,5),0,8,0);
        x = fi(zeros(4,1),0,8,0);
        header_nibbles(1) = fi(bitshift(plen, -4),0,8,0);
        header_nibbles(2) = fi(bitand(plen, 15),0,8,0);
        header_nibbles(3) = fi(bitor(2*cr, crc),0,8,0);
        tmp1 = fi(header_nibbles(1),0,4,0);
        tmp2 = fi(header_nibbles(2),0,4,0);
        tmp3 = fi(header_nibbles(3),0,4,0);
        header_nibbles(4) = fi(bitxor(bitxor(bitget(tmp1,1),bitget(tmp1,2)),bitxor(bitget(tmp1,3),bitget(tmp1,4))),0,8,0);
        x(1) = fi(bitxor(bitxor(bitxor(bitget(tmp1,4),bitget(tmp2,4)),bitxor(bitget(tmp2,2),bitget(tmp2,3))),bitget(tmp3,1)),0,8,0);
        x(2) = fi(bitxor(bitxor(bitxor(bitget(tmp1,3),bitget(tmp2,1)),bitxor(bitget(tmp2,4),bitget(tmp3,2))),bitget(tmp3,4)),0,8,0);
        x(3) = fi(bitxor(bitxor(bitxor(bitget(tmp1,2),bitget(tmp2,3)),bitxor(bitget(tmp2,1),bitget(tmp3,2))),bitxor(bitget(tmp3,3),bitget(tmp3,1))),0,8,0);
        x(4) = fi(bitxor(bitxor(bitxor(bitget(tmp1,1),bitget(tmp2,2)),bitxor(bitget(tmp3,1),bitget(tmp3,2))),bitxor(bitget(tmp3,3),bitget(tmp3,4))),0,8,0);
        header_nibbles(5) = fi(bitor(header_nibbles(5), bitshift(x(1),3)),0,8,0);
        header_nibbles(5) = fi(bitor(header_nibbles(5), bitshift(x(2),2)),0,8,0);
        header_nibbles(5) = fi(bitor(header_nibbles(5), bitshift(x(3),1)),0,8,0);
        header_nibbles(5) = fi(bitor(header_nibbles(5), x(4)),0,8,0);
        tmp_nibbles(1:5)=fi(header_nibbles,0,8,0);
        if idx<=fi(nibble_num,0,8,0)
            if fi(bitget(fi(idx,0,8,0),1),0,8,0)==fi(1,0,8,0)
                tmp_nibbles(idx+5)=fi(bitand(data_w(w_idx), 0xf),0,8,0);
            else
                tmp_nibbles(idx+5)=fi(bitshift(data_w(w_idx), -4),0,8,0);
                w_idx=fi(w_idx+1,0,8,0);
            end
            idx=fi(idx+1,0,8,0);
            nibbles=fi(zeros(1,16),0,8,0);
            nibbles_rdy=false;
        else
            nibbles=tmp_nibbles;
            nibbles_rdy=true;
        end
    else
        if idx<=fi(nibble_num,0,8,0)
            if fi(bitget(fi(idx,0,8,0),1),0,8,0)==fi(1,0,8,0)
                tmp_nibbles(idx)=fi(bitand(data_w(w_idx), 0xf),0,8,0);
            else
                tmp_nibbles(idx)=fi(bitshift(data_w(w_idx), -4),0,8,0);
                w_idx=fi(w_idx+1,0,8,0);
            end
            idx=fi(idx+1,0,8,0);
            nibbles=fi(zeros(1,16),0,8,0);
            nibbles_rdy=false;
        else
            nibbles=tmp_nibbles;
            nibbles_rdy=true;
        end
    end
else
    nibbles=fi(zeros(1,16),0,8,0);
    nibbles_rdy=false;
end

== matlab function Lora_os_all_16M64M_bw500sf12/LoRa_OSmod_CLK_SLOW/lorabb/Modulate/Symbol Generator ==
  data: modulate_nd output; data_symbols input; sym_num input; preamble_len input; symbol output; addr input; is_up output
function [modulate_nd,symbol,is_up] = fcn(data_symbols,sym_num,preamble_len,addr)
if addr==fi(0,0,16,0)
    symbol=fi(0,0,16,0);
    is_up=true;
    modulate_nd=false;
elseif addr<=fi(preamble_len,0,16,0)
    symbol=fi(0,0,16,0);
    is_up=true;
    modulate_nd=true;
elseif addr==fi(preamble_len+fi(1,0,16,0),0,16,0)
    symbol=fi(24,0,16,0);
    is_up=true;
    modulate_nd=true;
elseif addr==fi(preamble_len+fi(2,0,16,0),0,16,0)
    symbol=fi(32,0,16,0);
    is_up=true;
    modulate_nd=true;
elseif addr<=fi(preamble_len+fi(5,0,16,0),0,16,0)
    symbol=fi(0,0,16,0);
    is_up=false;
    modulate_nd=true;
elseif addr<=fi(preamble_len+fi(5,0,16,0)+fi(sym_num,0,16,0),0,16,0)
    symbol=fi(data_symbols(addr-preamble_len-5),0,16,0);
    is_up=true;
    modulate_nd=true;
else
    symbol=fi(0,0,16,0);
    is_up=true;
    modulate_nd=false;
end

== matlab function Lora_os_all_16M64M_bw500sf12/LoRa_OSmod_CLK_SLOW/lorabb/Encode/Interleave/interleave ==
  settings: fimath=fimath('RoundingMethod', 'Floor','OverflowAction', 'Wrap','ProductMode', 'FullPrecision', 'SumMode', 'FullPrecision')
  data: codewords input; codewords_rdy input; sym_num input; symbols_i output; sf input; ldr input; cr input; symbols_i_rdy output
function [symbols_i,symbols_i_rdy] = interleave(codewords,codewords_rdy,sym_num,sf,ldr,cr)
persistent p_idx...
           l_idx...
           b_idx...
           i_idx...
           ppm_num...
           packet...
           tmp_symbol...
           tmp_symbols_i
if isempty(p_idx)
    p_idx=fi(1,0,8,0);
end
if isempty(l_idx)
    l_idx=fi(1,0,8,0);
end
if isempty(b_idx)
    b_idx=fi(1,0,8,0);
end
if isempty(i_idx)
    i_idx=fi(0,0,8,0);
end
if isempty(ppm_num)
    ppm_num=fi(1,0,8,0);
end
if isempty(packet)
    packet=fi(zeros(1,16),0,8,0);
end
if isempty(tmp_symbol)
    tmp_symbol=fi(0,0,16,0);
end
if isempty(tmp_symbols_i)
    tmp_symbols_i=fi(zeros(1,64),0,16,0);
end

ppm = bitsliceget(fi(sf,0,8,0)-fi(ldr,0,8,0)-fi(ldr,0,8,0),8,1);
rdd = bitsliceget(fi(cr,0,8,0)+fi(4,0,8,0),8,1);
if codewords_rdy==true
    if p_idx<bitsliceget(fi(sf,0,8,0)-fi(1,0,8,0),8,1)
        packet(p_idx)=codewords(p_idx);
        if fi(p_idx,0,8,0)==bitsliceget(fi(sf,0,8,0)-fi(2,0,8,0),8,1)
            array=bitget(packet,l_idx);
            lsblocation=fi(l_idx,0,8,0);
            if lsblocation>bitsliceget(fi(sf,0,8,0)-fi(2,0,8,0),8,1)
                lsblocation=bitsliceget(fi(l_idx,0,8,0)+fi(2,0,8,0)-fi(sf,0,8,0),8,1);
            end
            if b_idx<lsblocation
                tmp_symbol=bitsliceget(tmp_symbol+tmp_symbol+fi(array(lsblocation-b_idx),0,16,0),16,1);
            elseif b_idx<fi(sf-1,0,8,0)
                tmp_symbol=bitsliceget(tmp_symbol+tmp_symbol+fi(array(sf-2+lsblocation-b_idx),0,16,0),16,1);
            end
            b_idx=fi(b_idx+1,0,8,0);
            if b_idx==bitsliceget(fi(sf,0,8,0)-fi(1,0,8,0),8,1)
                l_idx=fi(l_idx+1,0,8,0);
                b_idx=fi(1,0,8,0);
                i_idx=fi(i_idx+1,0,8,0);
                tmp_symbols_i(i_idx)=tmp_symbol;
                tmp_symbol=fi(0,0,16,0);
            end
            if l_idx==fi(9,0,8,0)
                p_idx=fi(p_idx+1,0,8,0);
                l_idx=fi(1,0,8,0);
            end
        else
            p_idx=fi(p_idx+1,0,8,0);
        end
        symbols_i_rdy=false;
        symbols_i=fi(zeros(1,64),0,16,0);
    elseif i_idx<fi(sym_num,0,8,0)
        packet(ppm_num)=codewords(p_idx);
        if ppm_num==ppm
            array=bitget(packet,l_idx);
            lsblocation=fi(l_idx,0,8,0);
            if lsblocation>ppm
                lsblocation=bitsliceget(fi(l_idx,0,8,0)-fi(ppm,0,8,0),8,1);
            end
            if b_idx<lsblocation
                tmp_symbol=bitsliceget(tmp_symbol+tmp_symbol+fi(array(lsblocation-b_idx),0,16,0),16,1);
                b_idx=fi(b_idx+1,0,8,0);
            elseif b_idx<=fi(ppm,0,8,0)
                tmp_symbol=bitsliceget(tmp_symbol+tmp_symbol+fi(array(ppm+lsblocation-b_idx),0,16,0),16,1);
            end
            b_idx=fi(b_idx+1,0,8,0);
            if b_idx==fi(ppm+1,0,8,0)
                l_idx=fi(l_idx+1,0,8,0);
                b_idx=fi(1,0,8,0);
                i_idx=fi(i_idx+1,0,8,0);
                tmp_symbols_i(i_idx)=tmp_symbol;
                tmp_symbol=fi(0,0,16,0);
            end
            if l_idx==fi(rdd+1,0,8,0)
                ppm_num=fi(1,0,8,0);
                p_idx=fi(p_idx+1,0,8,0);
                l_idx=fi(1,0,8,0);
            end
        else
            p_idx=fi(p_idx+1,0,8,0);
            ppm_num=fi(ppm_num+1,0,8,0);
        end
        symbols_i_rdy=false;
        symbols_i=fi(zeros(1,64),0,16,0);
    else
        symbols_i_rdy=true;
        symbols_i=tmp_symbols_i;
    end
else
    symbols_i_rdy=false;
    symbols_i=fi(zeros(1,64),0,16,0);
end

== matlab function Lora_os_all_16M64M_bw500sf12/LoRa_OSmod_CLK_SLOW/lorabb/Encode/Whiten/MATLAB Function ==
  data: data input; data_rdy input; sym_num input; plen input; sf input; data_w output; data_w_rdy output; cr input; ldr input; nibble_num output; crc input
function [data_w,data_w_rdy,nibble_num] = whiten(data, data_rdy, sym_num, plen, sf, cr, ldr, crc)
persistent idx...
           w_idx...
           dataw...
           tmp_data_w...
           reg
if isempty(idx)
    idx=fi(1,0,8,0);
end
if isempty(w_idx)
    w_idx=fi(1,0,8,0);
end
if isempty(dataw)
    dataw=fi(zeros(1,16),0,8,0); %生成待白化序列
end
if isempty(tmp_data_w)
    tmp_data_w=fi(zeros(1,16),0,8,0); %最后转为data_w
end
if isempty(reg)
    reg=fi(255,0,8,0); %原本的data_w
end

nibble_num = fi(sf-2+(sym_num-8)/(cr+4)*(sf-2*ldr),0,8,0);
if data_rdy==true
    if fi(idx,0,8,0) <= fi(plen+crc+crc,0,8,0)   %现在plen=4,2*crc是因为 若crc=1则有两个bit的checksum
        dataw(idx)=fi(data(idx),0,8,0);
        idx = fi(idx+1,0,8,0);
        dataw_rdy = false;
    elseif fi(2*idx,0,8,0)<=bitsliceget(nibble_num+fi(1,0,8,0),8,1)   %向上取整，所以nibble_num+1
        dataw(idx)=fi(255,0,8,0);
        idx = fi(idx+1,0,8,0);
        dataw_rdy = false;
    else
        idx = fi(length(dataw)+1,0,8,0);
        dataw_rdy = true;
    end
    if dataw_rdy==true  %待白化序列准备好了
        if w_idx<=fi(nibble_num,0,8,0)
            if fi(w_idx,0,8,0) <= fi(plen,0,8,0)
                tmp_data_w(w_idx) = bitxor(dataw(w_idx), reg);
                if reg<=fi(127,0,8,0)
                    tmp=reg;
                else
                    tmp=bitsliceget(reg-fi(128,0,8,0),8,1);
                end
                reg = bitxor(bitshift(tmp,1), fi(bitxor(bitget(reg,8), bitxor(bitget(reg,6), bitxor(bitget(reg,5), bitget(reg,4)))),0,8,0));
            else 
                tmp_data_w(w_idx) = dataw(w_idx);
            end
            w_idx = fi(w_idx+1,0,8,0);
            data_w = fi(zeros(1,16),0,8,0);
            data_w_rdy = false;
        else
            data_w = tmp_data_w;
            data_w_rdy=true;
        end
    else
        data_w = fi(zeros(1,16),0,8,0);
        data_w_rdy = false;
    end
else
    data_w = fi(zeros(1,16),0,8,0);
    data_w_rdy=false;
end

== matlab function Lora_os_all_16M64M_bw500sf12/LoRa_OSmod_CLK_SLOW/lorabb/Encode/Calc_sym_num/Calc_sym_num ==
  data: sym_num output; plen input; cr input; sf input; crc input; has_header input; ldr input
function sym_num = calc_sym_num(plen, cr, sf, crc, has_header,ldr)
    % calc_sym_num  Calculate number of symbols
    %
    % input:
    %     plen: Payload length 也可以传进来payload然后用length()函数
    % output:
    %     sym_num: Number of symbols
    if fi(2*plen+7+4*crc,0,8,0)<fi(sf+5*(1-has_header),0,8,0)
        tmp=fi(0,0,8,0);
    else
        tmp=fi((4+cr)*ceil((2*plen+7+4*crc-sf-5*(1-has_header))/(sf-2*ldr)),0,8,0);
        if fi(tmp*(sf-2*ldr),0,8,0)<fi((4+cr)*(2*plen+7+4*crc-sf-5*(1-has_header)),0,8,0)
            tmp=fi(tmp+fi(4+cr,0,8,0),0,8,0);
        end
    end
    sym_num =  bitsliceget(fi(tmp,0,8,0)+fi(8,0,8,0),8,1);
end

== matlab function Lora_os_all_16M64M_bw500sf12/LoRa_OSmod_CLK_SLOW/lorabb/Encode/Hamming/hamming ==
  data: sf input; codewords output; cr input; nibbles input; nibbles_rdy input; codewords_rdy output
function [codewords,codewords_rdy] = hamming(sf,cr,nibbles,nibbles_rdy)
% 未截断
    persistent idx ...
               tmp_codewords

    if isempty(idx)
        idx = fi(1,0,8,0);
    end
    if isempty(tmp_codewords)
        tmp_codewords = fi(zeros(1,16),0,8,0);
    end

    % 第一个是数据，第二个是是否有符号，第三个是数据位数，第四个是小数点位数。相当于uint8(0)
    if nibbles_rdy == true
        if idx <= fi(16,0,8,0)
            nibble = nibbles(idx);
            tmp = fi(nibble,0,8,0);
            codeword = fi(0,0,8,0);
            p1 = bitxor(bitget(tmp,1),bitxor(bitget(tmp,3),bitget(tmp,4))); % 1,3,4
            p2 = bitxor(bitget(tmp,1),bitxor(bitget(tmp,2),bitget(tmp,4))); % 1,2,4
            p3 = bitxor(bitget(tmp,1),bitxor(bitget(tmp,2),bitget(tmp,3))); % 1,2,3
            p4 = bitxor(bitxor(bitget(tmp,1),bitget(tmp,2)),bitxor(bitget(tmp,3),bitget(tmp,4))); % 1,2,3,4
            p5 = bitxor(bitget(tmp,2),bitxor(bitget(tmp,3),bitget(tmp,4))); % 2,3,4
            if idx <= sf - 2 % the first SF-2 nibbles use CR=4/8
                cr_tmp = fi(4,0,8,0);
            else 
                cr_tmp = fi(cr,0,8,0);
            end
            if cr_tmp == 1 % 4/5   % 或许用bit_shift来弄成乘法！
                codeword = bitor(fi(p4*16,0,8,0),tmp); % uint8()把大于255的数全部强制置为255，而小于255的部分则保持原样不变
            elseif cr_tmp == 2  % 4/6
                codeword = bitor(bitor(fi(p5*32,0,8,0),fi(p3*16,0,8,0)),tmp); % 冗余码生成 本质上就是简单加和
            elseif cr_tmp == 3  % 4/7
                codeword = bitor(bitor(fi(p2*64,0,8,0),fi(p5*32,0,8,0)),bitor(fi(p3*16,0,8,0),tmp));
            elseif cr_tmp == 4  % 4/8
                codeword = bitor(bitor(bitor(fi(p1*128,0,8,0),fi(p2*64,0,8,0)),bitor(fi(p5*32,0,8,0),fi(p3*16,0,8,0))),tmp);           
            end
            tmp_codewords(idx) = fi(codeword,0,8,0);
            idx=fi(idx+1,0,8,0);
            codewords=fi(zeros(1,16),0,8,0);
            codewords_rdy=false;
        else
            codewords = tmp_codewords;
            codewords_rdy=true;
        end
    else
        codewords=fi(zeros(1,16),0,8,0);  
        codewords_rdy=false;
    end
end
